simulink model "sis_PID"  (R2019b)
settings: Solver=VariableStepAuto  StartTime=0.0  StopTime=10.0  RelTol=1e-3
undefined symbols (not defined in the file): den_G1, den_G2, den_Rdo, den_Ri, den_Rpf, num_G1, num_G2, num_Rdo, num_Ri, num_Rpf
settings Model: Creator=edoardo  LastModifiedBy=edoardo

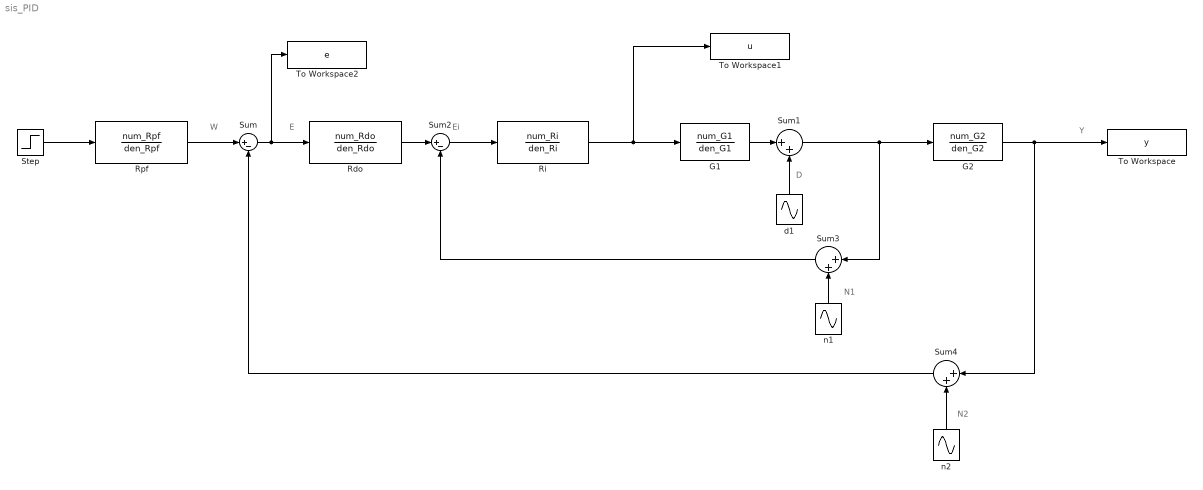
== system sis_PID ==
  note: W
  note: E
  note: Ei
  note: N1
  note: D
  note: Y
  note: N2
  "G1 " : TransferFcn  Numerator=num_G1  Denominator=den_G1
  G2 : TransferFcn  Numerator=num_G2  Denominator=den_G2
  Rdo : TransferFcn  Numerator=num_Rdo  Denominator=den_Rdo
  "Ri " : TransferFcn  Numerator=num_Ri  Denominator=den_Ri
  "Rpf " : TransferFcn  Numerator=num_Rpf  Denominator=den_Rpf
  Step : Step  Time=0  After=1.5  SampleTime=0
  Sum : Sum  Inputs=|+-
  Sum1 : Sum  Inputs=|++
  Sum2 : Sum  Inputs=|+-
  Sum3 : Sum  Inputs=|++
  Sum4 : Sum  Inputs=|++
  To Workspace : ToWorkspace  VariableName=y  SaveFormat=Timeseries  SampleTime=-1
  To Workspace1 : ToWorkspace  VariableName=u  SaveFormat=Timeseries  SampleTime=-1
  To Workspace2 : ToWorkspace  VariableName=e  SaveFormat=Timeseries  SampleTime=-1
  d1 : Sin  Amplitude=3  SampleTime=0
  n1 : Sin  Amplitude=0.02  Frequency=8000  SampleTime=0
  n2 : Sin  Amplitude=0.02  Frequency=8000  SampleTime=0
  wires:
  Sum3/1 -> Sum2/2
  "Ri "/1 -> To Workspace1/1, "G1 "/1
  n2/1 -> Sum4/2
  Sum1/1 -> Sum3/1, G2/1
  n1/1 -> Sum3/2
  d1/1 -> Sum1/2
  Sum/1 -> Rdo/1, To Workspace2/1
  Sum4/1 -> Sum/2
  "G1 "/1 -> Sum1/1
  G2/1 -> Sum4/1, To Workspace/1
  Sum2/1 -> "Ri "/1
  Rdo/1 -> Sum2/1
  Step/1 -> "Rpf "/1
  "Rpf "/1 -> Sum/1
